simulink model "SBR_sep_model"  (R2025a)
settings: Solver=VariableStepAuto  StartTime=0.0  StopTime=10  RelTol=1e-3
libraries: cstblocks x3
settings Model: Creator=banom  LastModifiedBy=banom

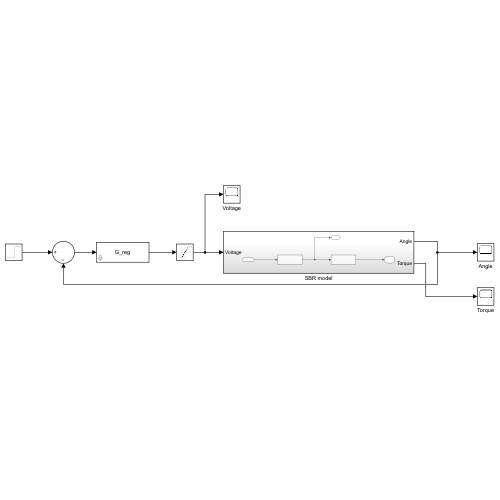
[thumbnail: Simulink's stored preview of the top-level diagram]
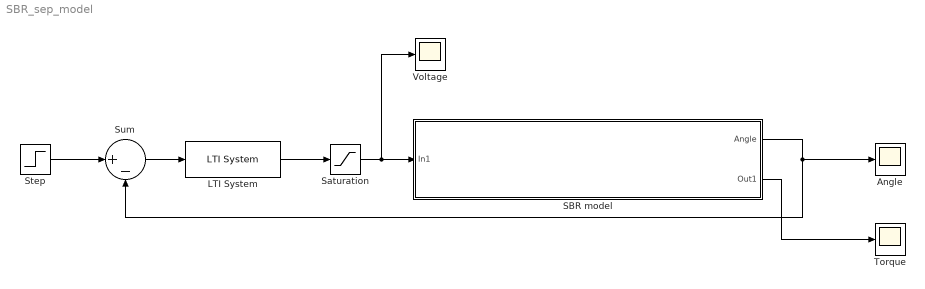
== system SBR_sep_model ==
  Angle : Scope
      settings: ActiveDisplayYMinimum=-0.46164593543265464  ActiveDisplayYMaximum=4.1548134188938928
  LTI System : cstblocks/LTI System  sys=G_reg  IC=[]  PadeOrder=0
  SBR model : Subsystem
  Saturation : Saturate  UpperLimit=6  LowerLimit=-6
  Step : Step  Time=0  Before=pi/9  After=pi  SampleTime=0
  Sum : Sum  Inputs=|+-
  Torque : Scope
      settings: ActiveDisplayYMinimum=-102.15741988718821  ActiveDisplayYMaximum=106.02623705174824  DataLoggingVariableName=ScopeData2
  Voltage : Scope
      settings: ActiveDisplayYMinimum=-8.5488662645580646  ActiveDisplayYMaximum=8.1982817308323828
  wires:
  SBR model/1(Angle) -> Sum/2, Angle/1
  Step/1 -> Sum/1
  Sum/1 -> LTI System/1
  SBR model/2(Out1) -> Torque/1
  LTI System/1 -> Saturation/1
  Saturation/1 -> Voltage/1, SBR model/1(In1)

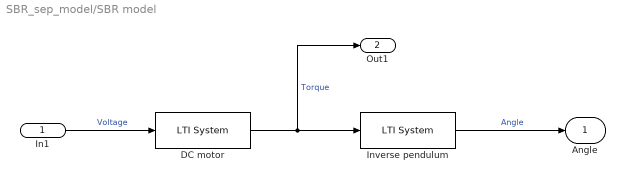
== system SBR_sep_model/SBR model ==
  In1 : Inport
  DC motor : cstblocks/LTI System  sys=G_volt_torq  IC=[]  PadeOrder=0
  Inverse pendulum : cstblocks/LTI System  sys=G_torq_ang  IC=[]  PadeOrder=0
  Angle : Outport
  Out1 : Outport  Port=2
  wires:
  DC motor/1 -> Out1/1, Inverse pendulum/1  "Torque"
  Inverse pendulum/1 -> Angle/1  "Angle"
  In1/1 -> DC motor/1  "Voltage"
